simulink model "sampleModel1863"  (R2023a)
settings: Solver=VariableStepAuto  StartTime=0.0  StopTime=10.0  RelTol=1e-3
libraries: hdlsllib x4, simulink x2
settings Model: Creator=user1  LastModifiedBy=user1

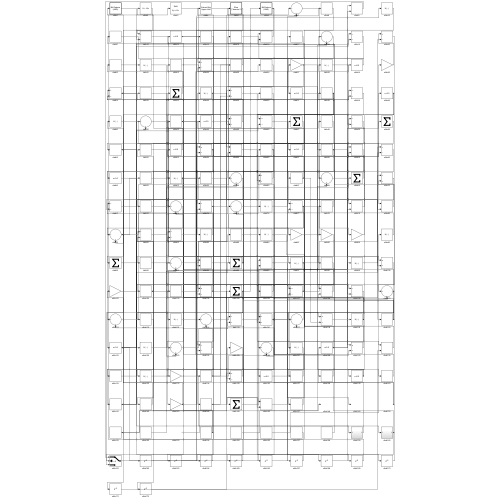
[thumbnail: Simulink's stored preview of the top-level diagram]
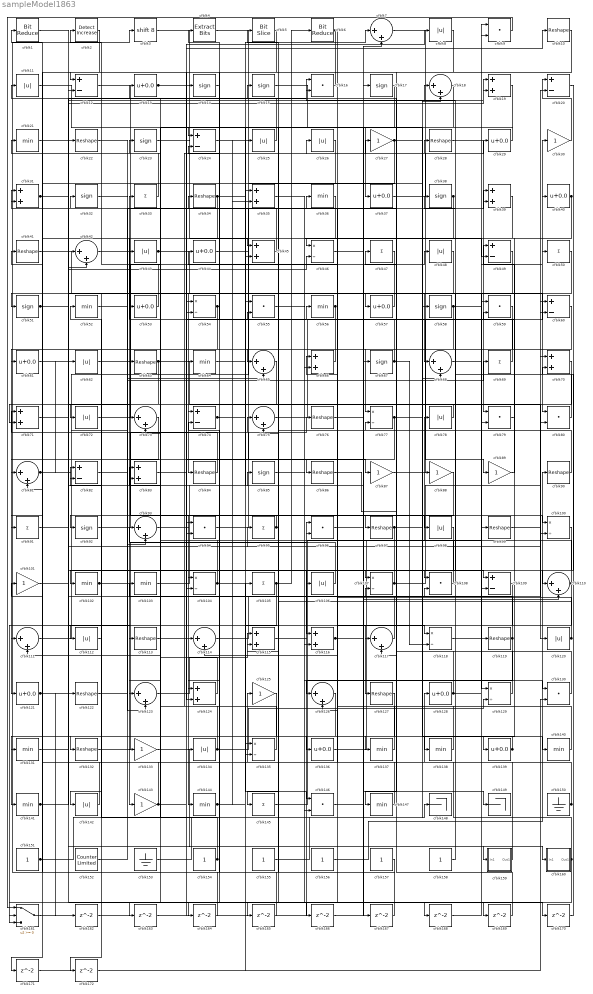
== system sampleModel1863 ==
  cfblk1 : hdlsllib/Logic and Bit Operations/Bit Reduce  mode=AND
  cfblk{10,22,28,34,41,63,76,84,86,90,97,99,113,119,122,127,132} (17 alike) : Reshape
  cfblk{46,54,77,100,104,107,118,129,135} (9 alike) : Product  Inputs=*/  RndMeth=Zero  SaturateOnIntegerOverflow=on
  cfblk{27,30,87..89,101,125,133,143} (9 alike) : Gain
  cfblk{21,36,52,56,64,102..103,131,137..138,140..141,144,147} (14 alike) : MinMax
  cfblk{33,47,50,69,91,95,105,145} (8 alike) : Sum  Inputs=+
  cfblk{8,11,25..26,43,48,62,72,78,98,106,112,120,134,142} (15 alike) : Abs  SaturateOnIntegerOverflow=off
  cfblk{9,16,55,59,79..80,94,96,108,130,146} (11 alike) : DotProduct  OutDataTypeStr=Inherit: Inherit via internal rule
  cfblk{12,20,24,49,60,74,82,109} (8 alike) : Sum  Inputs=+-
  cfblk{7,18,42,65,68,73,75,81,93,110..111,114,117,123,126} (15 alike) : Sum  Inputs=|++
  cfblk{19,31,35,39,45,66,70..71,83,115..116,124} (12 alike) : Sum
  cfblk{13,29,37,40,44,53,57,61,121,128,136,139} (12 alike) : Bias  Bias=0.0  SaturateOnIntegerOverflow=off
  cfblk{14..15,17,23,32,38,51,58,67,85,92} (11 alike) : Signum
  cfblk148 : Terminator
  cfblk149 : Terminator
  cfblk150 : Ground
  cfblk{151,154..158} (6 alike) : Constant  SampleTime=-1
  cfblk152 : hdlsllib/Sources/Counter Limited  uplimit=7  tsamp=-1
  cfblk153 : Ground
  cfblk159 : Subsystem
      settings: LibrarySourceBlock=|
      | hdlsllib/Ports &
      | Subsystems/Subsystem
  cfblk160 : Subsystem
      settings: LibrarySourceBlock=|
      | hdlsllib/Ports &
      | Subsystems/Subsystem
  cfblk161 : Switch  SaturateOnIntegerOverflow=off  InputSameDT=off
  cfblk{162..172} (11 alike) : Delay  SampleTime=1
  cfblk2 : simulink/Logic and Bit Operations/Detect Increase  vinit=0.0  OutDataTypeStr=boolean
      settings: LibrarySourceBlock=|
      | hdlsllib/Logic and Bit
      | Operations/Detect
      | Increase
  cfblk3 : ArithShift  BitShiftNumber=8
  cfblk4 : simulink/Logic and Bit Operations/Extract Bits  bitsToExtract=Upper half  numBits=8  bitIdxRange=[0 7]  outScalingMode=Preserve fixed-point scaling
      settings: LibrarySourceBlock=|
      | hdlsllib/Logic and Bit
      | Operations/Extract Bits
  cfblk5 : hdlsllib/Logic and Bit Operations/Bit Slice  lidx=7  ridx=0
  cfblk6 : hdlsllib/Logic and Bit Operations/Bit Reduce  mode=AND
  wires:
  cfblk48/1 -> cfblk84/1
  cfblk87/1 -> cfblk30/1
  cfblk81/1 -> cfblk62/1, cfblk65/2
  cfblk135/1 -> cfblk26/1
  cfblk126/1 -> cfblk52/1
  cfblk153/1 -> cfblk148/1
  cfblk4/1 -> cfblk86/1
  cfblk83/1 -> cfblk56/1
  cfblk157/1 -> cfblk3/1
  cfblk121/1 -> cfblk95/1, cfblk16/2, cfblk160/1(In1), cfblk162/1
  cfblk28/1 -> cfblk79/1
  cfblk62/1 -> cfblk97/1
  cfblk111/1 -> cfblk39/1
  cfblk7/1 -> cfblk89/1
  cfblk49/1 -> cfblk102/1
  cfblk3/1 -> cfblk45/1
  cfblk161/1 -> cfblk96/1
  cfblk29/1 -> cfblk24/1
  cfblk70/1 -> cfblk74/1
  cfblk72/1 -> cfblk48/1
  cfblk92/1 -> cfblk75/1
  cfblk31/1 -> cfblk19/2, cfblk168/1
  cfblk78/1 -> cfblk72/1
  cfblk97/1 -> cfblk132/1, cfblk18/2
  cfblk95/1 -> cfblk92/1, cfblk5/1
  cfblk57/1 -> cfblk51/1
  cfblk12/1 -> cfblk87/1
  cfblk86/1 -> cfblk147/1
  cfblk90/1 -> cfblk32/1
  cfblk115/1 -> cfblk79/2
  cfblk18/1 -> cfblk145/1
  cfblk91/1 -> cfblk122/1
  cfblk156/1 -> cfblk90/1
  cfblk43/1 -> cfblk80/1, cfblk100/2
  cfblk127/1 -> cfblk141/1
  cfblk103/1 -> cfblk17/1
  cfblk74/1 -> cfblk7/1, cfblk104/1
  cfblk136/1 -> cfblk78/1
  cfblk68/1 -> cfblk9/1
  cfblk37/1 -> cfblk29/1
  cfblk160/1(Out1) -> cfblk128/1, cfblk161/2
  cfblk145/1 -> cfblk9/2
  cfblk15/1 -> cfblk88/1
  cfblk77/1 -> cfblk140/1, cfblk104/2, cfblk126/2
  cfblk137/1 -> cfblk44/1
  cfblk34/1 -> cfblk143/1, cfblk80/2
  cfblk85/1 -> cfblk130/1
  cfblk118/1 -> cfblk119/1
  cfblk54/1 -> cfblk121/1, cfblk124/1
  cfblk41/1 -> cfblk129/1
  cfblk106/1 -> cfblk93/1
  cfblk66/1 -> cfblk65/1
  cfblk63/1 -> cfblk120/1, cfblk98/1, cfblk71/2
  cfblk132/1 -> cfblk96/2
  cfblk104/1 -> cfblk23/1, cfblk146/2
  cfblk33/1 -> cfblk21/1
  cfblk75/1 -> cfblk40/1
  cfblk10/1 -> cfblk81/1
  cfblk134/1 -> cfblk129/2, cfblk25/1, cfblk111/2
  cfblk152/1 -> cfblk93/2
  cfblk159/1(Out1) -> cfblk125/1
  cfblk9/1 -> cfblk161/1
  cfblk17/1 -> cfblk37/1
  cfblk133/1 -> cfblk159/1(In1)
  cfblk42/1 -> cfblk144/1
  cfblk30/1 -> cfblk20/1
  cfblk84/1 -> cfblk71/1
  cfblk22/1 -> cfblk107/1
  cfblk110/1 -> cfblk47/1, cfblk117/2, cfblk166/1
  cfblk56/1 -> cfblk61/1, cfblk165/1
  cfblk19/1 -> cfblk63/1
  cfblk13/1 -> cfblk55/1, cfblk10/1
  cfblk8/1 -> cfblk137/1
  cfblk99/1 -> cfblk60/1
  cfblk21/1 -> cfblk22/1
  cfblk67/1 -> cfblk33/1, cfblk118/2
  cfblk59/1 -> cfblk77/1
  cfblk158/1 -> cfblk38/1
  cfblk98/1 -> cfblk116/1
  cfblk61/1 -> cfblk113/1
  cfblk147/1 -> cfblk36/1
  cfblk16/1 -> cfblk12/1
  cfblk47/1 -> cfblk64/1
  cfblk11/1 -> cfblk67/1
  cfblk114/1 -> cfblk70/1
  cfblk141/1 -> cfblk42/1, cfblk46/2, cfblk85/1
  cfblk94/1 -> cfblk76/1
  cfblk27/1 -> cfblk81/2, cfblk109/1
  cfblk113/1 -> cfblk14/1
  cfblk151/1 -> cfblk135/1, cfblk94/1
  cfblk71/1 -> cfblk73/1
  cfblk39/1 -> cfblk57/1
  cfblk76/1 -> cfblk28/1
  cfblk44/1 -> cfblk68/1
  cfblk58/1 -> cfblk100/1, cfblk163/1
  cfblk125/1 -> cfblk131/1
  cfblk53/1 -> cfblk11/1
  cfblk102/1 -> cfblk20/2, cfblk82/2
  cfblk108/1 -> cfblk31/1
  cfblk116/1 -> cfblk118/1, cfblk170/1
  cfblk117/1 -> cfblk83/1
  cfblk80/1 -> cfblk16/1
  cfblk93/1 -> cfblk35/1
  cfblk109/1 -> cfblk127/1
  cfblk51/1 -> cfblk19/1, cfblk109/2
  cfblk79/1 -> cfblk49/1
  cfblk107/1 -> cfblk60/2, cfblk106/1
  cfblk25/1 -> cfblk2/1
  cfblk105/1 -> cfblk112/1, cfblk6/1, cfblk161/3
  cfblk100/1 -> cfblk123/1
  cfblk65/1 -> cfblk91/1
  cfblk155/1 -> cfblk68/2
  cfblk40/1 -> cfblk139/1, cfblk94/2
  cfblk142/1 -> cfblk101/1
  cfblk122/1 -> cfblk34/1
  cfblk89/1 -> cfblk59/2
  cfblk131/1 -> cfblk107/2
  cfblk2/1 -> cfblk12/2
  cfblk138/1 -> cfblk114/2
  cfblk120/1 -> cfblk66/1, cfblk18/1, cfblk55/2
  cfblk1/1 -> cfblk54/2
  cfblk24/1 -> cfblk58/1
  cfblk129/1 -> cfblk15/1
  cfblk124/1 -> cfblk73/2
  cfblk154/1 -> cfblk43/1, cfblk82/1
  cfblk140/1 -> cfblk103/1
  cfblk26/1 -> cfblk45/2
  cfblk32/1 -> cfblk39/2
  cfblk23/1 -> cfblk27/1
  cfblk20/1 -> cfblk110/1
  cfblk69/1 -> cfblk4/1
  cfblk123/1 -> cfblk115/1
  cfblk139/1 -> cfblk138/1, cfblk133/1
  cfblk130/1 -> cfblk31/2
  cfblk146/1 -> cfblk110/2
  cfblk60/1 -> cfblk142/1
  cfblk101/1 -> cfblk42/2
  cfblk38/1 -> cfblk66/2, cfblk111/1, cfblk116/2
  cfblk128/1 -> cfblk99/1, cfblk50/1, cfblk53/1
  cfblk88/1 -> cfblk135/2
  cfblk52/1 -> cfblk123/2
  cfblk35/1 -> cfblk49/2
  cfblk82/1 -> cfblk69/1
  cfblk64/1 -> cfblk117/1
  cfblk6/1 -> cfblk126/1, cfblk124/2
  cfblk46/1 -> cfblk149/1
  cfblk143/1 -> cfblk8/1, cfblk41/1
  cfblk150/1 -> cfblk115/2, cfblk108/2
  cfblk119/1 -> cfblk83/2, cfblk13/1, cfblk136/1
  cfblk50/1 -> cfblk108/1
  cfblk144/1 -> cfblk146/1, cfblk35/2
  cfblk5/1 -> cfblk134/1
  cfblk36/1 -> cfblk46/1
  cfblk45/1 -> cfblk24/2
  cfblk162/1 -> cfblk54/1
  cfblk163/1 -> cfblk114/1
  cfblk14/1 -> cfblk164/1
  cfblk164/1 -> cfblk1/1
  cfblk165/1 -> cfblk74/2
  cfblk166/1 -> cfblk7/2
  cfblk96/1 -> cfblk167/1
  cfblk167/1 -> cfblk75/2
  cfblk168/1 -> cfblk59/1
  cfblk55/1 -> cfblk169/1
  cfblk169/1 -> cfblk77/2
  cfblk170/1 -> cfblk70/2
  cfblk73/1 -> cfblk171/1
  cfblk171/1 -> cfblk130/2
  cfblk112/1 -> cfblk172/1
  cfblk172/1 -> cfblk105/1

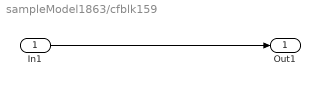
== system sampleModel1863/cfblk159 ==
  In1 : Inport
  Out1 : Outport
  wires:
  In1/1 -> Out1/1

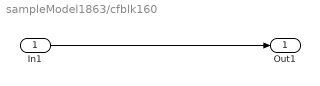
== system sampleModel1863/cfblk160 ==
  In1 : Inport
  Out1 : Outport
  wires:
  In1/1 -> Out1/1
